simulink model "Actuator_Control"  (R2022b)
settings: configuration reference "csMultiInstance" (kept outside this file)
model workspace (MATLAB code in the model file):
  | localDD_Actuator_Control;
undefined symbols (not defined in the file): Kp
libraries: simulink x1
Description:
  | This model implements the hydraulic actuator control of the helicopter flight control software.
settings Model: DataDictionary=DD_Actuator_Control.sldd  EnableAccessToBaseWorkspace=off  ParameterArgumentNames=Kp,Ki,Kd,N  Creator=The MathWorks, Inc.  LastModifiedBy=The MathWorks, Inc.
settings ConfigSetRef: SourceName=csMultiInstance

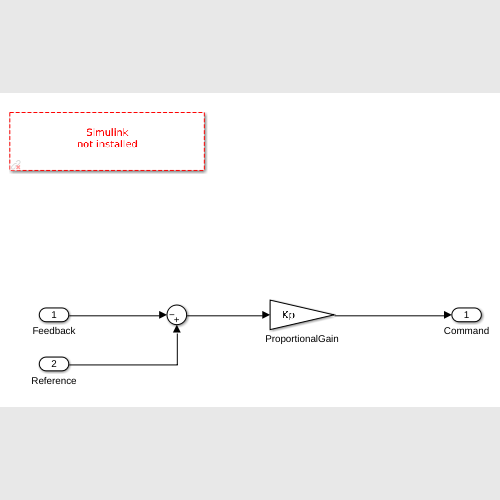
[thumbnail: Simulink's stored preview of the top-level diagram]
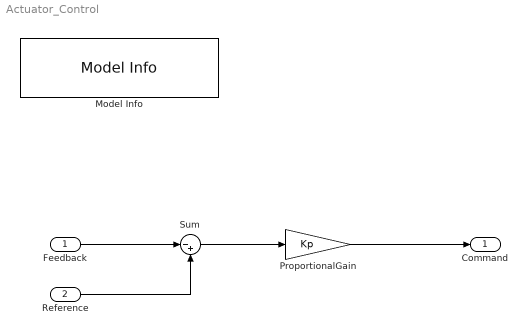
== system Actuator_Control ==
  Feedback : Inport  OutMin=-0.1  OutMax=0.1  OutDataTypeStr=double  PortDimensions=1  SampleTime=0.001
  Reference : Inport  Port=2  OutMin=-0.1  OutMax=0.1  OutDataTypeStr=double  PortDimensions=1  SampleTime=0.001
  Model Info : simulink/Model-Wide Utilities/Model Info  Frame=on  DisplayStringWithTags=|  HorizontalTextAlignment=Center  LeftAlignmentValue=0.5
      | Model Name: %<ModelName>
      | Model Version: %<ModelVersion>
      | Last Modified: %<LastModificationDate>
  ProportionalGain : Gain  Gain=Kp
  Sum : Sum  Inputs=|-+
  Command : Outport  VectorParamsAs1DForOutWhenUnconnected=off
  wires:
  Feedback/1 -> Sum/1
  Reference/1 -> Sum/2
  Sum/1 -> ProportionalGain/1
  ProportionalGain/1 -> Command/1
